simulink model "Quad_Nonlinear_PID_Roll_Pitch"  (R2020a)
settings: Solver=ode4  StartTime=0.0  StopTime=15  FixedStep=0.02  RelTol=1e-3
InitFcn:
  | QuadParameter
values from neighbouring files (symbols this model uses):
  AHRS_RCP = AHRS(251:end, :)    [PS_I.m]    (also in PS_II.m = AHRS(271:end, :); PS_III.m)
  KD_Pitch = 10^savedata{1}(3)*2.1    [load_data.m]
  KD_Roll = 10^savedata{1}(3)*2.1    [load_data.m]
  KI_Pitch = 10^savedata{1}(2)*500    [load_data.m]
  KI_Roll = 10^savedata{1}(2)*500    [load_data.m]
  KP_Pitch = 10^savedata{1}(1)*2    [load_data.m]
  KP_Roll = 10^savedata{1}(1)*2    [load_data.m]
undefined symbols (not defined in the file or in its folder): b, d_cg, g, h_cg, J_R, J_xx, J_yy, m2, m_tot, magnitude, miu_k, r_y
libraries: simulink x3
settings Model: OrderedModelArguments=off  Creator=Ali  LastModifiedBy=Ali

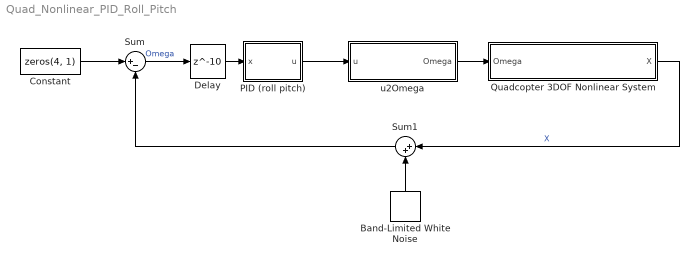
== system Quad_Nonlinear_PID_Roll_Pitch ==
  Band-Limited White Noise : simulink/Sources/Band-Limited White Noise  Cov=[0.005]  Ts=0.2  seed=[23341]
  Constant : Constant  Value=zeros(4, 1)
  Delay : Delay  DelayLength=10
  PID (roll pitch) : Subsystem
  Quadcopter 3DOF Nonlinear System : Subsystem  TreatAsAtomicUnit=on
  Sum : Sum  Inputs=|+-
  Sum1 : Sum  Inputs=|++
  u2Omega : Subsystem
  wires:
  Sum/1 -> Delay/1  "Omega"
  PID (roll pitch)/1(u) -> u2Omega/1(u)
  u2Omega/1(Omega) -> Quadcopter 3DOF Nonlinear System/1(Omega)
  Constant/1 -> Sum/1
  Quadcopter 3DOF Nonlinear System/1(X) -> Sum1/1  "X"
  Sum1/1 -> Sum/2
  Band-Limited White Noise/1 -> Sum1/2
  Delay/1 -> PID (roll pitch)/1(x)

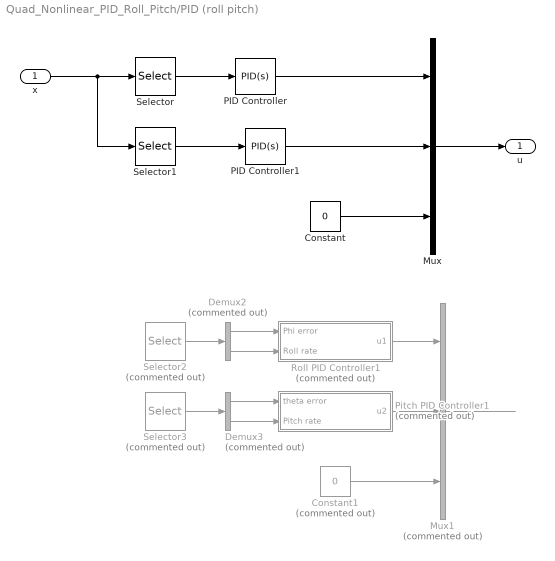
== system Quad_Nonlinear_PID_Roll_Pitch/PID (roll pitch) ==
  x : Inport
  Constant : Constant  Value=0
  Constant1 : Constant  Commented=on  Value=0
  Demux2 : Demux  Commented=on  Outputs=2
  Demux3 : Demux  Commented=on  Outputs=2
  Mux : Mux  Inputs=3
  Mux1 : Mux  Commented=on  Inputs=3
  PID Controller : simulink/Continuous/PID Controller  Controller=PID  Form=Parallel  TimeDomain=Continuous-time  UseExternalTs=off  SampleTime=-1  IntegratorMethod=Forward Euler  FilterMethod=Forward Euler  ControllerParametersSource=internal  P=1  I=1  D=0  UseFilter=on  N=100  TunerSelectOption=Transfer Function Based (PID Tuner App)  InitialConditionSource=internal  InitialConditionForIntegrator=0  InitialConditionForFilter=0  DifferentiatorICPrevScaledInput=0  ExternalReset=none  TrackingMode=off  Kt=1  LimitOutput=off  UpperSaturationLimit=inf  LowerSaturationLimit=-inf  LinearizeAsGain=on  AntiWindupMode=none  Kb=1  POutMin=[]  POutMax=[]  IOutMin=[]  IOutMax=[]  DOutMin=[]  DOutMax=[]  NOutMin=[]  NOutMax=[]  SumOutMin=[]  SumOutMax=[]  SaturationOutMin=[]  SaturationOutMax=[]  PParamMin=[]  PParamMax=[]  IParamMin=[]  IParamMax=[]  DParamMin=[]  DParamMax=[]  NParamMin=[]  NParamMax=[]  KbParamMin=[]  KbParamMax=[]  KtParamMin=[]  KtParamMax=[]  KbOutMin=[]  KbOutMax=[]  KtOutMin=[]  KtOutMax=[]  IntegratorOutMin=[]  IntegratorOutMax=[]  FilterOutMin=[]  FilterOutMax=[]  SumI1OutMin=[]  SumI1OutMax=[]  SumI2OutMin=[]  SumI2OutMax=[]  SumI3OutMin=[]  SumI3OutMax=[]  SumI4OutMin=[]  SumI4OutMax=[]  SumDOutMin=[]  SumDOutMax=[]  DifferentiatorOutMin=[]  DifferentiatorOutMax=[]  FilterDiffOutCoefMin=[]  FilterDiffOutCoefMax=[]  ReciprocalOutMin=[]  ReciprocalOutMax=[]  SumDenOutMin=[]  SumDenOutMax=[]  SumNumOutMin=[]  SumNumOutMax=[]  DivideOutMin=[]  DivideOutMax=[]  UdiffTsProdOutMin=[]  UdiffTsProdOutMax=[]  NTsProdOutMin=[]  NTsProdOutMax=[]  UintegralTsProdOutMin=[]  UintegralTsProdOutMax=[]  UngainTsProdOutMin=[]  UngainTsProdOutMax=[]  IntegratorContinuousStateAttributes=''  IntegratorStateMustResolveToSignalObject=off  IntegratorRTWStateStorageClass=Auto  FilterContinuousStateAttributes=''  FilterStateMustResolveToSignalObject=off  FilterRTWStateStorageClass=Auto  ParallelPVariant=InternalParameters  IdealPVariant=Disabled  IVariant=InternalParameters  DVariant=InternalParameters  IntegratorVariant=Continuous  SatVariant=Disabled  AWVariant=Passthrough  PCopyVariant=Disabled  TRVariant=Disabled  FdbkBlocksVariant=Forward  IdealPFdbkVariant=Disabled  SatFdbkVariant=Disabled  DerivativeFilterVariant=ContFilter  NVariant=InternalParameters  NCopyVariant=Disabled  FilterICVariant=InternalICsFilter  IntegratorICVariant=InternalICs  ExternalResetVariant=Disabled  TRSumVariant=Passthrough  SumFdbkVariant=Disabled  SumVariant=Sum_PID  TsampFilterVariant=InternalTs  TsampNgainVariant=Passthrough  TsampIntegralVariant=Passthrough
  PID Controller1 : simulink/Continuous/PID Controller  Controller=PID  Form=Parallel  TimeDomain=Continuous-time  UseExternalTs=off  SampleTime=-1  IntegratorMethod=Forward Euler  FilterMethod=Forward Euler  ControllerParametersSource=internal  P=1  I=1  D=0  UseFilter=on  N=100  TunerSelectOption=Transfer Function Based (PID Tuner App)  InitialConditionSource=internal  InitialConditionForIntegrator=0  InitialConditionForFilter=0  DifferentiatorICPrevScaledInput=0  ExternalReset=none  TrackingMode=off  Kt=1  LimitOutput=off  UpperSaturationLimit=inf  LowerSaturationLimit=-inf  LinearizeAsGain=on  AntiWindupMode=none  Kb=1  POutMin=[]  POutMax=[]  IOutMin=[]  IOutMax=[]  DOutMin=[]  DOutMax=[]  NOutMin=[]  NOutMax=[]  SumOutMin=[]  SumOutMax=[]  SaturationOutMin=[]  SaturationOutMax=[]  PParamMin=[]  PParamMax=[]  IParamMin=[]  IParamMax=[]  DParamMin=[]  DParamMax=[]  NParamMin=[]  NParamMax=[]  KbParamMin=[]  KbParamMax=[]  KtParamMin=[]  KtParamMax=[]  KbOutMin=[]  KbOutMax=[]  KtOutMin=[]  KtOutMax=[]  IntegratorOutMin=[]  IntegratorOutMax=[]  FilterOutMin=[]  FilterOutMax=[]  SumI1OutMin=[]  SumI1OutMax=[]  SumI2OutMin=[]  SumI2OutMax=[]  SumI3OutMin=[]  SumI3OutMax=[]  SumI4OutMin=[]  SumI4OutMax=[]  SumDOutMin=[]  SumDOutMax=[]  DifferentiatorOutMin=[]  DifferentiatorOutMax=[]  FilterDiffOutCoefMin=[]  FilterDiffOutCoefMax=[]  ReciprocalOutMin=[]  ReciprocalOutMax=[]  SumDenOutMin=[]  SumDenOutMax=[]  SumNumOutMin=[]  SumNumOutMax=[]  DivideOutMin=[]  DivideOutMax=[]  UdiffTsProdOutMin=[]  UdiffTsProdOutMax=[]  NTsProdOutMin=[]  NTsProdOutMax=[]  UintegralTsProdOutMin=[]  UintegralTsProdOutMax=[]  UngainTsProdOutMin=[]  UngainTsProdOutMax=[]  IntegratorContinuousStateAttributes=''  IntegratorStateMustResolveToSignalObject=off  IntegratorRTWStateStorageClass=Auto  FilterContinuousStateAttributes=''  FilterStateMustResolveToSignalObject=off  FilterRTWStateStorageClass=Auto  ParallelPVariant=InternalParameters  IdealPVariant=Disabled  IVariant=InternalParameters  DVariant=InternalParameters  IntegratorVariant=Continuous  SatVariant=Disabled  AWVariant=Passthrough  PCopyVariant=Disabled  TRVariant=Disabled  FdbkBlocksVariant=Forward  IdealPFdbkVariant=Disabled  SatFdbkVariant=Disabled  DerivativeFilterVariant=ContFilter  NVariant=InternalParameters  NCopyVariant=Disabled  FilterICVariant=InternalICsFilter  IntegratorICVariant=InternalICs  ExternalResetVariant=Disabled  TRSumVariant=Passthrough  SumFdbkVariant=Disabled  SumVariant=Sum_PID  TsampFilterVariant=InternalTs  TsampNgainVariant=Passthrough  TsampIntegralVariant=Passthrough
  Pitch PID Controller1 : Subsystem  Commented=on  VariantControl=Choice
  Roll PID Controller1 : Subsystem  Commented=on  VariantControl=Choice
  Selector : Selector  InputPortWidth=4  IndexOptions=Index vector (dialog)  Indices=[1]  OutputSizes=1
  Selector1 : Selector  InputPortWidth=4  IndexOptions=Index vector (dialog)  Indices=[2]  OutputSizes=1
  Selector2 : Selector  Commented=on  InputPortWidth=4  IndexOptions=Index vector (dialog)  Indices=[1 3]  OutputSizes=1
  Selector3 : Selector  Commented=on  InputPortWidth=4  IndexOptions=Index vector (dialog)  Indices=[2 4]  OutputSizes=1
  u : Outport
  wires:
  x/1 -> Selector1/1, Selector/1
  Mux/1 -> u/1
  Constant/1 -> Mux/3
  Roll PID Controller1/1(u1) -> Mux1/1
  Demux3/1 -> Pitch PID Controller1/1(theta error)
  Mux1/1 -> ?
  Demux3/2 -> Pitch PID Controller1/2(Pitch rate)
  ? -> Selector3/1
  Demux2/2 -> Roll PID Controller1/2(Roll rate)
  Selector3/1 -> Demux3/1
  Constant1/1 -> Mux1/3
  ? -> Selector2/1
  Selector2/1 -> Demux2/1
  Pitch PID Controller1/1(u2) -> Mux1/2
  Demux2/1 -> Roll PID Controller1/1(Phi error)
  Selector/1 -> PID Controller/1
  PID Controller/1 -> Mux/1
  Selector1/1 -> PID Controller1/1
  PID Controller1/1 -> Mux/2

== system Quad_Nonlinear_PID_Roll_Pitch/Quadcopter 3DOF Nonlinear System ==
  Omega : Inport
  Integrator : Integrator  InitialCondition=AHRS_RCP(1, :)
  Quad System : Subsystem
  Saturation : Saturate  UpperLimit=[0.7871 inf 0.7871 inf]  LowerLimit=[-0.5867 -inf -0.5867 -inf]
  X : Outport
  wires:
  Integrator/1 -> Quad System/1(X), Saturation/1  "X"
  Quad System/1(dot(X)) -> Integrator/1  "dot(X)"
  Omega/1 -> Quad System/2(Omega)
  Saturation/1 -> X/1

== system Quad_Nonlinear_PID_Roll_Pitch/u2Omega ==
  u : Inport
  MATLAB Function : MATLAB Function  TreatAsAtomicUnit=on
  Mux1 : Mux
  Omega : Outport
  wires:
  MATLAB Function/2(omega_2) -> Mux1/2
  u/1 -> MATLAB Function/1(u)
  MATLAB Function/3(omega_3) -> Mux1/3
  MATLAB Function/1(omega_1) -> Mux1/1
  MATLAB Function/4(omega_4) -> Mux1/4
  Mux1/1 -> Omega/1

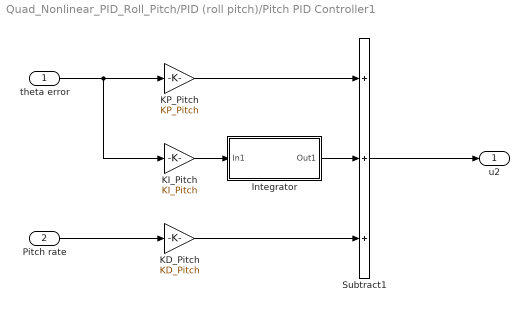
== system Quad_Nonlinear_PID_Roll_Pitch/PID (roll pitch)/Pitch PID Controller1 ==
  theta error : Inport
  Pitch rate : Inport  Port=2
  Integrator : Subsystem
  KD_Pitch : Gain  Gain=KD_Pitch
  KI_Pitch : Gain  Gain=KI_Pitch
  KP_Pitch : Gain  Gain=KP_Pitch
  Subtract1 : Sum  Inputs=+++
  u2 : Outport
  wires:
  Integrator/1(Out1) -> Subtract1/2
  KI_Pitch/1 -> Integrator/1(In1)
  KD_Pitch/1 -> Subtract1/3
  Subtract1/1 -> u2/1
  KP_Pitch/1 -> Subtract1/1
  Pitch rate/1 -> KD_Pitch/1
  theta error/1 -> KI_Pitch/1, KP_Pitch/1

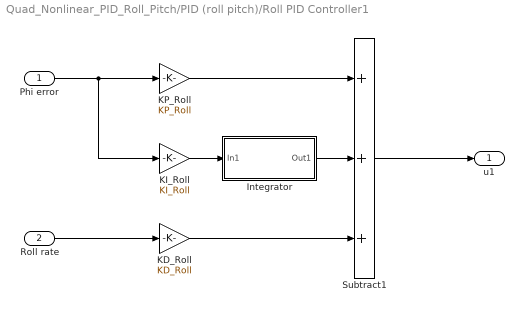
== system Quad_Nonlinear_PID_Roll_Pitch/PID (roll pitch)/Roll PID Controller1 ==
  Phi error : Inport
  Roll rate : Inport  Port=2
  Integrator : Subsystem
  KD_Roll : Gain  Gain=KD_Roll
  KI_Roll : Gain  Gain=KI_Roll
  KP_Roll : Gain  Gain=KP_Roll
  Subtract1 : Sum  Inputs=+++
  u1 : Outport
  wires:
  Integrator/1(Out1) -> Subtract1/2
  KI_Roll/1 -> Integrator/1(In1)
  KD_Roll/1 -> Subtract1/3
  Subtract1/1 -> u1/1
  KP_Roll/1 -> Subtract1/1
  Roll rate/1 -> KD_Roll/1
  Phi error/1 -> KI_Roll/1, KP_Roll/1

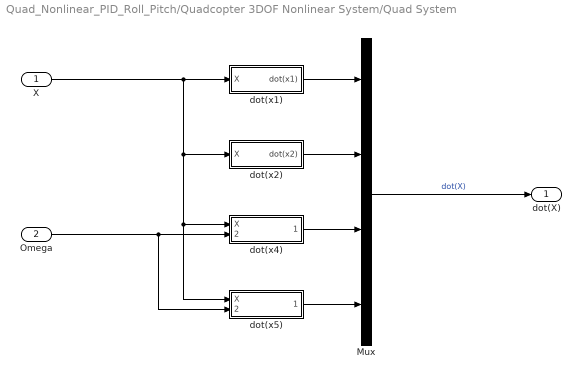
== system Quad_Nonlinear_PID_Roll_Pitch/Quadcopter 3DOF Nonlinear System/Quad System ==
  X : Inport
  Omega : Inport  Port=2
  Mux : Mux
  dot(x1) : Subsystem
  dot(x2) : Subsystem
  dot(x4) : Subsystem
  dot(x5) : Subsystem
  dot(X) : Outport
  wires:
  Mux/1 -> dot(X)/1  "dot(X)"
  X/1 -> dot(x5)/1(X), dot(x4)/1(X), dot(x2)/1(X), dot(x1)/1(X)
  Omega/1 -> dot(x5)/2(Omega), dot(x4)/2(Omega)
  dot(x2)/1(dot(x2)) -> Mux/2
  dot(x1)/1(dot(x1)) -> Mux/1
  dot(x4)/1(dot(x4)) -> Mux/3
  dot(x5)/1(dot(x5)) -> Mux/4

== system Quad_Nonlinear_PID_Roll_Pitch/PID (roll pitch)/Pitch PID Controller1/Integrator ==
  In1 : Inport
  Clock : Clock
  Integrator1 : Integrator
  Starter : Subsystem
  Switch : Switch  Criteria=u2 > Threshold  Threshold=5
  Out1 : Outport
  wires:
  Integrator1/1 -> Out1/1
  Clock/1 -> Switch/2
  In1/1 -> Switch/1
  Starter/1(start_pulse) -> Switch/3
  Switch/1 -> Integrator1/1

== system Quad_Nonlinear_PID_Roll_Pitch/PID (roll pitch)/Roll PID Controller1/Integrator ==
  In1 : Inport
  Clock : Clock
  Integrator1 : Integrator
  Starter : Subsystem
  Switch : Switch  Criteria=u2 > Threshold  Threshold=5
  Out1 : Outport
  wires:
  Integrator1/1 -> Out1/1
  Clock/1 -> Switch/2
  In1/1 -> Switch/1
  Starter/1(start_pulse) -> Switch/3
  Switch/1 -> Integrator1/1

== system Quad_Nonlinear_PID_Roll_Pitch/Quadcopter 3DOF Nonlinear System/Quad System/dot(x1) ==
  X : Inport
  1 : Subsystem
  Add : Sum  Inputs=+++
  Subsystem : Subsystem
  Subsystem1 : Subsystem
  dot(x1) : Outport
  wires:
  X/1 -> Subsystem1/1(X), Subsystem/1(X), 1/1(X)  "X"
  Subsystem1/1(x4) -> Add/3
  Subsystem/1(x6cos(x1)tan(x2)) -> Add/2
  Add/1 -> dot(x1)/1
  1/1(x5sin(x1)tan(x2)) -> Add/1

== system Quad_Nonlinear_PID_Roll_Pitch/Quadcopter 3DOF Nonlinear System/Quad System/dot(x2) ==
  X : Inport
  1 : Subsystem
  dot(x2) : Outport
  wires:
  X/1 -> 1/1(X)  "X"
  1/1(x5cos(x1)) -> dot(x2)/1

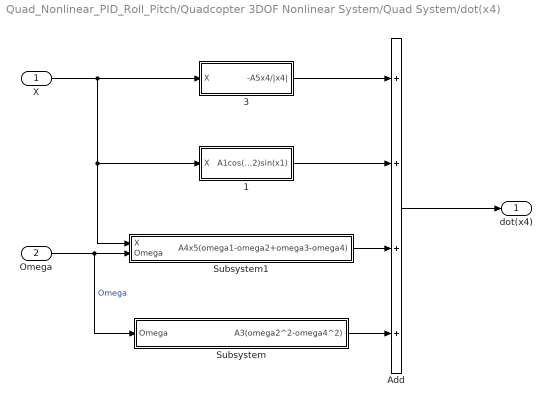
== system Quad_Nonlinear_PID_Roll_Pitch/Quadcopter 3DOF Nonlinear System/Quad System/dot(x4) ==
  X : Inport
  Omega : Inport  Port=2
  1 : Subsystem
  3 : Subsystem
  Add : Sum  Inputs=++++
  Subsystem : Subsystem
  Subsystem1 : Subsystem
  dot(x4) : Outport
  wires:
  X/1 -> Subsystem1/1(X), 1/1(X), 3/1(X)
  Omega/1 -> Subsystem/1(Omega), Subsystem1/2(Omega)  "Omega"
  Add/1 -> dot(x4)/1
  3/1("-A5x4/|x4| ") -> Add/1
  1/1(A1cos(x2)sin(x1)) -> Add/2
  Subsystem1/1(A4x5(omega1-omega2+omega3-omega4)) -> Add/3
  Subsystem/1(A3(omega2^2-omega4^2)) -> Add/4

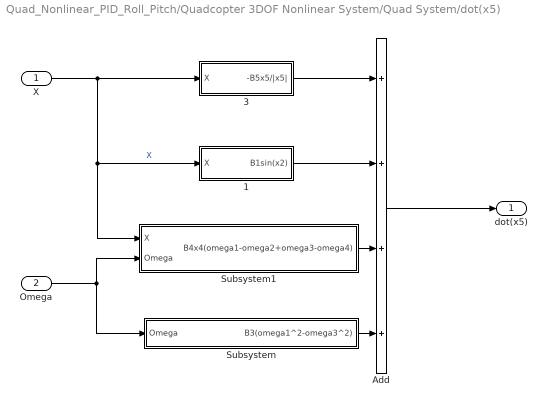
== system Quad_Nonlinear_PID_Roll_Pitch/Quadcopter 3DOF Nonlinear System/Quad System/dot(x5) ==
  X : Inport
  Omega : Inport  Port=2
  1 : Subsystem
  3 : Subsystem
  Add : Sum  Inputs=++++
  Subsystem : Subsystem
  Subsystem1 : Subsystem
  dot(x5) : Outport
  wires:
  X/1 -> Subsystem1/1(X), 1/1(X), 3/1(X)  "X"
  Omega/1 -> Subsystem/1(Omega), Subsystem1/2(Omega)
  Add/1 -> dot(x5)/1
  3/1("-B5x5/|x5| ") -> Add/1
  1/1(B1sin(x2)) -> Add/2
  Subsystem/1(B3(omega1^2-omega3^2)) -> Add/4
  Subsystem1/1(B4x4(omega1-omega2+omega3-omega4)) -> Add/3

== system Quad_Nonlinear_PID_Roll_Pitch/PID (roll pitch)/Pitch PID Controller1/Integrator/Starter ==
  Add : Sum
  Step : Step  After=140
  Step1 : Step  Time=2  After=-30
  start_pulse : Outport
  wires:
  Add/1 -> start_pulse/1
  Step/1 -> Add/1
  Step1/1 -> Add/2

== system Quad_Nonlinear_PID_Roll_Pitch/PID (roll pitch)/Roll PID Controller1/Integrator/Starter ==
  Add : Sum
  Step : Step  After=140
  Step1 : Step  Time=2  After=-30
  start_pulse : Outport
  wires:
  Add/1 -> start_pulse/1
  Step/1 -> Add/1
  Step1/1 -> Add/2

== system Quad_Nonlinear_PID_Roll_Pitch/Quadcopter 3DOF Nonlinear System/Quad System/dot(x1)/1 ==
  X : Inport
  Demux : Demux  Outputs=3
  Selector : Selector  InputPortWidth=4  IndexOptions=Index vector (dialog)  Indices=[1 2 4]  OutputSizes=1
  Subsystem : Subsystem
  x5sin(x1)tan(x2) : Outport
  wires:
  X/1 -> Selector/1  "x"
  Subsystem/1(x5sin(x1)tan(x2)) -> x5sin(x1)tan(x2)/1
  Selector/1 -> Demux/1
  Demux/1 -> Subsystem/1(x1)  "x1"
  Demux/2 -> Subsystem/2(x2)  "x2"
  Demux/3 -> Subsystem/3(x5)  "x5"

== system Quad_Nonlinear_PID_Roll_Pitch/Quadcopter 3DOF Nonlinear System/Quad System/dot(x1)/Subsystem ==
  X : Inport
  Demux : Demux  Outputs=2
  Selector : Selector  InputPortWidth=4  IndexOptions=Index vector (dialog)  Indices=[1 2]  OutputSizes=1
  Subsystem1 : Subsystem
  x6cos(x1)tan(x2) : Outport
  wires:
  Subsystem1/1(x6cos(x1)tan(x2)) -> x6cos(x1)tan(x2)/1  "x6cos(x1)tan(x2)"
  X/1 -> Selector/1  "X"
  Demux/1 -> Subsystem1/1(x1)
  Demux/2 -> Subsystem1/2(x2)
  Selector/1 -> Demux/1

== system Quad_Nonlinear_PID_Roll_Pitch/Quadcopter 3DOF Nonlinear System/Quad System/dot(x1)/Subsystem1 ==
  X : Inport
  Selector : Selector  InputPortWidth=4  IndexOptions=Index vector (dialog)  Indices=[3]  OutputSizes=1
  x4 : Outport
  wires:
  Selector/1 -> x4/1
  X/1 -> Selector/1

== system Quad_Nonlinear_PID_Roll_Pitch/Quadcopter 3DOF Nonlinear System/Quad System/dot(x2)/1 ==
  X : Inport
  Demux : Demux  Outputs=2
  Selector : Selector  InputPortWidth=4  IndexOptions=Index vector (dialog)  Indices=[1 4]  OutputSizes=1
  Subsystem : Subsystem
  x5cos(x1) : Outport
  wires:
  Subsystem/1(Out1) -> x5cos(x1)/1
  Demux/1 -> Subsystem/1(x1)
  Demux/2 -> Subsystem/2(x5)
  Selector/1 -> Demux/1
  X/1 -> Selector/1  "x"

== system Quad_Nonlinear_PID_Roll_Pitch/Quadcopter 3DOF Nonlinear System/Quad System/dot(x4)/1 ==
  X : Inport
  Demux : Demux  Outputs=2
  Selector : Selector  InputPortWidth=4  IndexOptions=Index vector (dialog)  Indices=[1 2]  OutputSizes=1
  Subsystem : Subsystem
  A1cos(x2)sin(x1) : Outport
  wires:
  Subsystem/1(A1cos(x2)sin(x1)) -> A1cos(x2)sin(x1)/1
  Demux/2 -> Subsystem/2(x2)
  Demux/1 -> Subsystem/1(x1)
  Selector/1 -> Demux/1
  X/1 -> Selector/1  "x"

== system Quad_Nonlinear_PID_Roll_Pitch/Quadcopter 3DOF Nonlinear System/Quad System/dot(x4)/3 ==
  X : Inport
  Selector : Selector  InputPortWidth=4  IndexOptions=Index vector (dialog)  Indices=[3]  OutputSizes=1
  Subsystem : Subsystem
  "-A5x4/|x4| " : Outport
  wires:
  Subsystem/1("-A5x4/|x4| ") -> "-A5x4/|x4| "/1
  Selector/1 -> Subsystem/1(x4)
  X/1 -> Selector/1  "x"

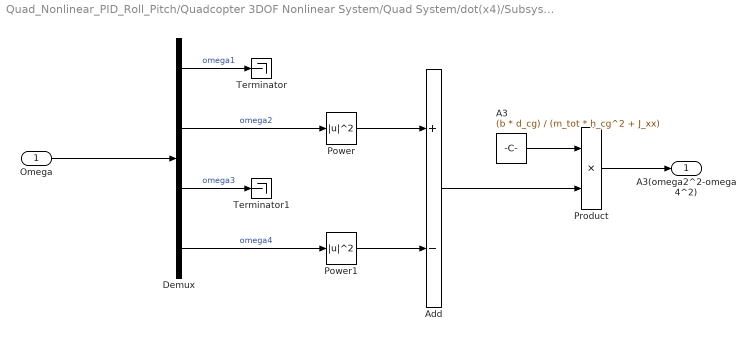
== system Quad_Nonlinear_PID_Roll_Pitch/Quadcopter 3DOF Nonlinear System/Quad System/dot(x4)/Subsystem ==
  Omega : Inport
  A3 : Constant  Value=(b * d_cg) / (m_tot * h_cg^2 + J_xx)
  Add : Sum  Inputs=+-
  Demux : Demux
  Power : Math  Operator=magnitude^2  SaturateOnIntegerOverflow=on
  Power1 : Math  Operator=magnitude^2  SaturateOnIntegerOverflow=on
  Product : Product
  Terminator : Terminator
  Terminator1 : Terminator
  A3(omega2^2-omega4^2) : Outport
  wires:
  Product/1 -> A3(omega2^2-omega4^2)/1
  Power1/1 -> Add/2
  Demux/2 -> Power/1  "omega2"
  Demux/4 -> Power1/1  "omega4"
  Add/1 -> Product/2
  Power/1 -> Add/1
  A3/1 -> Product/1
  Omega/1 -> Demux/1
  Demux/3 -> Terminator1/1  "omega3"
  Demux/1 -> Terminator/1  "omega1"

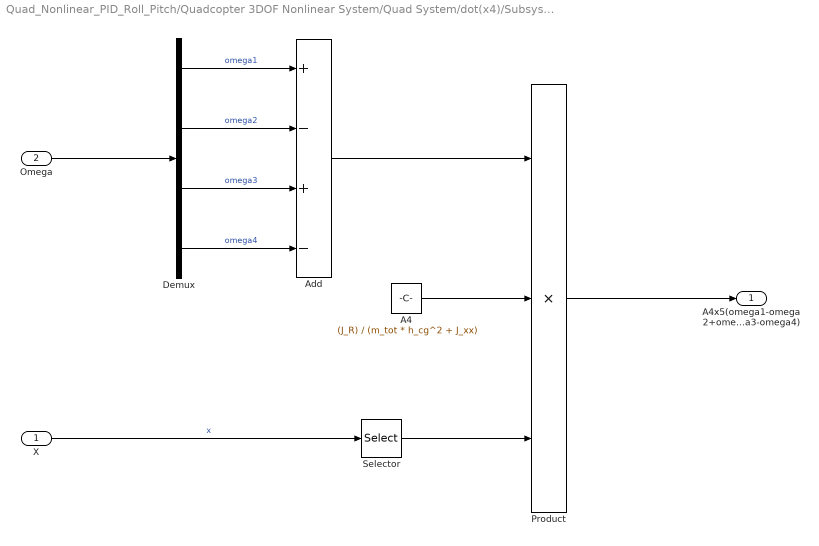
== system Quad_Nonlinear_PID_Roll_Pitch/Quadcopter 3DOF Nonlinear System/Quad System/dot(x4)/Subsystem1 ==
  X : Inport
  Omega : Inport  Port=2
  A4 : Constant  Value=(J_R) / (m_tot * h_cg^2 + J_xx)
  Add : Sum  Inputs=+-+-
  Demux : Demux
  Product : Product  Inputs=3
  Selector : Selector  InputPortWidth=4  IndexOptions=Index vector (dialog)  Indices=[4]  OutputSizes=1
  A4x5(omega1-omega2+omega3-omega4) : Outport
  wires:
  Omega/1 -> Demux/1
  Demux/1 -> Add/1  "omega1"
  Demux/2 -> Add/2  "omega2"
  Demux/3 -> Add/3  "omega3"
  Demux/4 -> Add/4  "omega4"
  Add/1 -> Product/1
  A4/1 -> Product/2
  Product/1 -> A4x5(omega1-omega2+omega3-omega4)/1
  Selector/1 -> Product/3
  X/1 -> Selector/1  "x"

== system Quad_Nonlinear_PID_Roll_Pitch/Quadcopter 3DOF Nonlinear System/Quad System/dot(x5)/1 ==
  X : Inport
  Selector : Selector  InputPortWidth=4  IndexOptions=Index vector (dialog)  Indices=[2]  OutputSizes=1
  Subsystem : Subsystem
  B1sin(x2) : Outport
  wires:
  Subsystem/1(B1sin(x2)) -> B1sin(x2)/1
  Selector/1 -> Subsystem/1(x2)
  X/1 -> Selector/1  "x"

== system Quad_Nonlinear_PID_Roll_Pitch/Quadcopter 3DOF Nonlinear System/Quad System/dot(x5)/3 ==
  X : Inport
  Selector : Selector  InputPortWidth=4  IndexOptions=Index vector (dialog)  Indices=[4]  OutputSizes=1
  Subsystem : Subsystem
  "-B5x5/|x5| " : Outport
  wires:
  Subsystem/1("-B5x5/|x5| ") -> "-B5x5/|x5| "/1
  X/1 -> Selector/1  "x"
  Selector/1 -> Subsystem/1(x5)

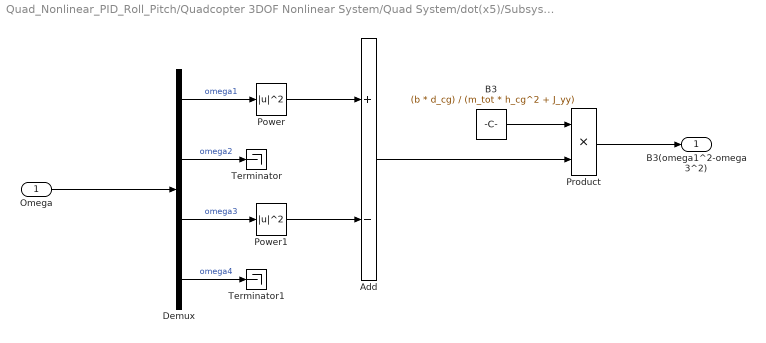
== system Quad_Nonlinear_PID_Roll_Pitch/Quadcopter 3DOF Nonlinear System/Quad System/dot(x5)/Subsystem ==
  Omega : Inport
  Add : Sum  Inputs=+-
  B3 : Constant  Value=(b * d_cg) / (m_tot * h_cg^2 + J_yy)
  Demux : Demux
  Power : Math  Operator=magnitude^2  SaturateOnIntegerOverflow=on
  Power1 : Math  Operator=magnitude^2  SaturateOnIntegerOverflow=on
  Product : Product
  Terminator : Terminator
  Terminator1 : Terminator
  B3(omega1^2-omega3^2) : Outport
  wires:
  Product/1 -> B3(omega1^2-omega3^2)/1
  Power1/1 -> Add/2
  Add/1 -> Product/2
  Power/1 -> Add/1
  B3/1 -> Product/1
  Omega/1 -> Demux/1
  Demux/3 -> Power1/1  "omega3"
  Demux/1 -> Power/1  "omega1"
  Demux/2 -> Terminator/1  "omega2"
  Demux/4 -> Terminator1/1  "omega4"

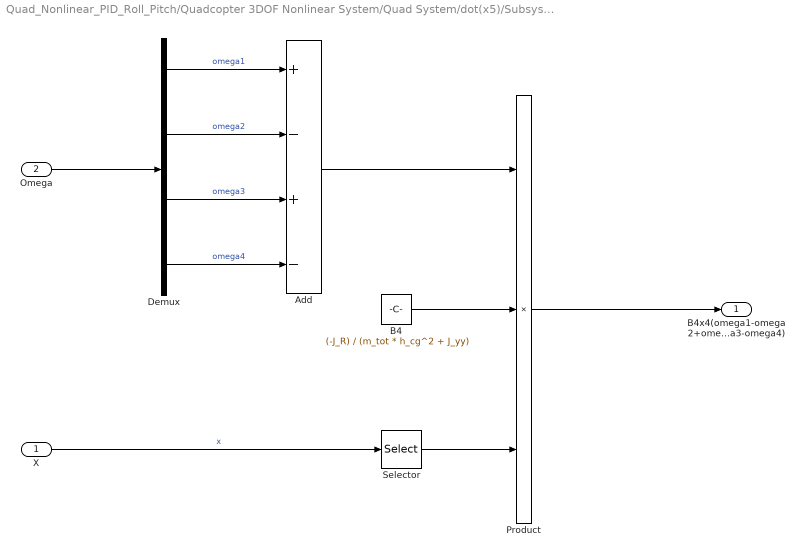
== system Quad_Nonlinear_PID_Roll_Pitch/Quadcopter 3DOF Nonlinear System/Quad System/dot(x5)/Subsystem1 ==
  X : Inport
  Omega : Inport  Port=2
  Add : Sum  Inputs=+-+-
  B4 : Constant  Value=(-J_R) / (m_tot * h_cg^2 + J_yy)
  Demux : Demux
  Product : Product  Inputs=3
  Selector : Selector  InputPortWidth=4  IndexOptions=Index vector (dialog)  Indices=[3]  OutputSizes=1
  B4x4(omega1-omega2+omega3-omega4) : Outport
  wires:
  Omega/1 -> Demux/1
  Demux/1 -> Add/1  "omega1"
  Demux/2 -> Add/2  "omega2"
  Demux/3 -> Add/3  "omega3"
  Demux/4 -> Add/4  "omega4"
  Add/1 -> Product/1
  B4/1 -> Product/2
  Product/1 -> B4x4(omega1-omega2+omega3-omega4)/1
  X/1 -> Selector/1  "x"
  Selector/1 -> Product/3

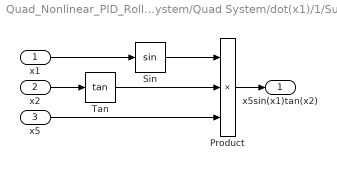
== system Quad_Nonlinear_PID_Roll_Pitch/Quadcopter 3DOF Nonlinear System/Quad System/dot(x1)/1/Subsystem ==
  x1 : Inport
  x2 : Inport  Port=2
  x5 : Inport  Port=3
  Product : Product  Inputs=3
  Sin : Trigonometry
  Tan : Trigonometry  Operator=tan
  x5sin(x1)tan(x2) : Outport
  wires:
  Sin/1 -> Product/1
  x5/1 -> Product/3
  Product/1 -> x5sin(x1)tan(x2)/1
  x1/1 -> Sin/1
  x2/1 -> Tan/1
  Tan/1 -> Product/2

== system Quad_Nonlinear_PID_Roll_Pitch/Quadcopter 3DOF Nonlinear System/Quad System/dot(x1)/Subsystem/Subsystem1 ==
  x1 : Inport
  x2 : Inport  Port=2
  Cos : Trigonometry  Operator=cos
  Product1 : Product
  Tan : Trigonometry  Operator=tan
  x6cos(x1)tan(x2) : Outport
  wires:
  x1/1 -> Cos/1
  Cos/1 -> Product1/1
  x2/1 -> Tan/1
  Product1/1 -> x6cos(x1)tan(x2)/1
  Tan/1 -> Product1/2

== system Quad_Nonlinear_PID_Roll_Pitch/Quadcopter 3DOF Nonlinear System/Quad System/dot(x2)/1/Subsystem ==
  x1 : Inport
  x5 : Inport  Port=2
  Cos : Trigonometry  Operator=cos
  Product : Product
  Out1 : Outport
  wires:
  Cos/1 -> Product/1
  Product/1 -> Out1/1
  x1/1 -> Cos/1
  x5/1 -> Product/2

== system Quad_Nonlinear_PID_Roll_Pitch/Quadcopter 3DOF Nonlinear System/Quad System/dot(x4)/1/Subsystem ==
  x1 : Inport
  x2 : Inport  Port=2
  A1 : Constant  Value=(h_cg * g * m_tot) / (m_tot * h_cg^2 + J_xx)
  Cos : Trigonometry  Operator=cos
  Product : Product  Inputs=3
  Sin : Trigonometry
  A1cos(x2)sin(x1) : Outport
  wires:
  Sin/1 -> Product/1
  Product/1 -> A1cos(x2)sin(x1)/1
  x1/1 -> Sin/1
  x2/1 -> Cos/1
  Cos/1 -> Product/2
  A1/1 -> Product/3

== system Quad_Nonlinear_PID_Roll_Pitch/Quadcopter 3DOF Nonlinear System/Quad System/dot(x4)/3/Subsystem ==
  x4 : Inport
  A5 : Constant  Value=(J_R) / (m_tot * h_cg^2 + J_xx)
  Gain : Gain  Gain=-1
  Switch : Switch  Criteria=u2 > Threshold
  "-A5x4/|x4| " : Outport
  wires:
  Switch/1 -> "-A5x4/|x4| "/1
  A5/1 -> Switch/3, Gain/1
  x4/1 -> Switch/2
  Gain/1 -> Switch/1

== system Quad_Nonlinear_PID_Roll_Pitch/Quadcopter 3DOF Nonlinear System/Quad System/dot(x5)/1/Subsystem ==
  x2 : Inport
  B1 : Constant  Value=(h_cg * g * m_tot) / (m_tot * h_cg^2 + J_yy)
  Product : Product
  Sin : Trigonometry
  B1sin(x2) : Outport
  wires:
  Product/1 -> B1sin(x2)/1
  x2/1 -> Sin/1
  B1/1 -> Product/2
  Sin/1 -> Product/1

== system Quad_Nonlinear_PID_Roll_Pitch/Quadcopter 3DOF Nonlinear System/Quad System/dot(x5)/3/Subsystem ==
  x5 : Inport
  B5 : Constant  Value=(m2 * g * miu_k * r_y) / (m_tot * h_cg^2 + J_yy)
  Gain : Gain  Gain=-1
  Switch : Switch  Criteria=u2 > Threshold
  "-B5x5/|x5| " : Outport
  wires:
  Switch/1 -> "-B5x5/|x5| "/1
  B5/1 -> Switch/3, Gain/1
  x5/1 -> Switch/2
  Gain/1 -> Switch/1

== matlab function Quad_Nonlinear_PID_Roll_Pitch/u2Omega/MATLAB Function ==
  data: u input size=3; omega_1 output size=1; omega_2 output size=1; omega_3 output size=1; omega_4 output size=1
function [omega_1, omega_2, omega_3, omega_4] = fcn(u)
u1 = u(1);
u2 = u(2);
u3 = u(3);
% control effort
u4 = ones(1, length(u1)) * 4 * rpm2rad_sec(2000)^2;
% calculate omega
if (u4 + u3 + 2 * u2) / 4 > 0
    omega_1 = sqrt((u4 + u3 + 2 * u2) / 4);
else
    omega_1 = 0;
end
if (u4 + u3 - 2 * u2) / 4 > 0
    omega_3 = sqrt((u4 + u3 - 2 * u2) / 4);
else
    omega_3 = 0;
end
if (u4 - u3 + 2 * u1) / 4 > 0
    omega_2 = sqrt((u4 - u3 + 2 * u1) / 4);
else
    omega_2 = 0;
end
if (u4 - u3 - 2 * u1) / 4 > 0
    omega_4 = sqrt((u4 - u3 - 2 * u1) / 4);
else
    omega_4 = 0;
end
end
%% functions
% rpm to rad/sec
function rad = rpm2rad_sec(rpm)
rad = rpm / 60 * 2 * pi;
end
